simulink model "inverse_dynamic_control"  (R2017b)
settings: Solver=VariableStepAuto  StartTime=0.0  StopTime=3  RelTol=1e-3
InitFcn:
  | stop_time_as_str = get_param(gcs, 'StopTime');
  | stopTime = str2double(stop_time_as_str);
values from neighbouring files (symbols this model uses):
  KD = 50    [centralized_control_design.m]
  KP = 200    [centralized_control_design.m]
  max_torques = [56 97 52 10 10 10]    [centralized_control_design.m]
  min_torques = -[56 97 52 10 10 10]    [centralized_control_design.m]
libraries: roblocks x4
settings Model: Creator=jan  LastModifiedBy=jan.rosell

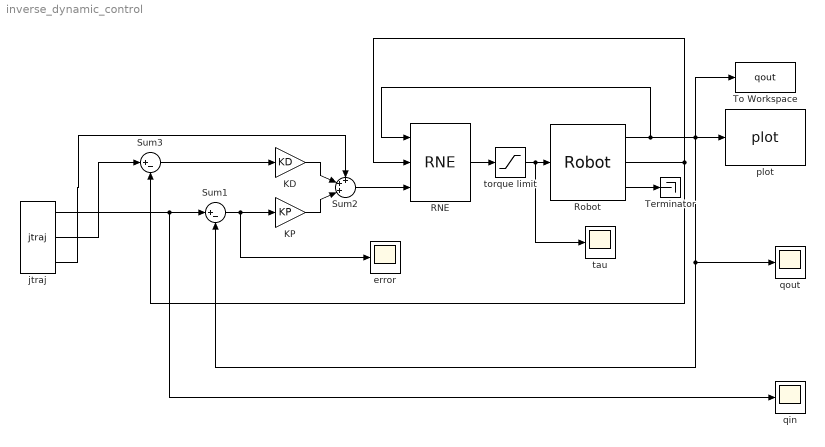
== system inverse_dynamic_control ==
  KD : Gain  Gain=KD
  KP : Gain  Gain=KP
  RNE : roblocks/Arm/RNE  robot=p560.nofriction  grav=[0 0 9.81]
  Robot : roblocks/Arm/Robot  robot=p560.nofriction  q0=[0 0 0 0 0 0]
  Sum1 : Sum  Inputs=|+-
  Sum2 : Sum  Inputs=+++|
  Sum3 : Sum  Inputs=|+-
  Terminator : Terminator
  To Workspace : ToWorkspace  VariableName=qout  SaveFormat=Timeseries  SampleTime=-1
  error : Scope
  jtraj : roblocks/Toolbox/jtraj  q0=[0 0 0 0 0 0]  qf=[pi/4 pi/2 -pi/2 0 0 0]  tmax=stopTime  ts=0.02
  plot : roblocks/Arm/plot  robot=p560  fps=10  holdplot=on
  qin : Scope
  qout : Scope
  tau : Scope
  torque limit : Saturate  UpperLimit=max_torques  LowerLimit=min_torques
  wires:
  Robot/3 -> Terminator/1
  Sum1/1 -> error/1, KP/1
  jtraj/1 -> qin/1, Sum1/1
  torque limit/1 -> tau/1, Robot/1
  RNE/1 -> torque limit/1
  Sum2/1 -> RNE/3
  Robot/1 -> RNE/1, To Workspace/1, plot/1, qout/1, Sum1/2
  Robot/2 -> Sum3/2, RNE/2
  KP/1 -> Sum2/3
  KD/1 -> Sum2/2
  jtraj/3 -> Sum2/1
  Sum3/1 -> KD/1
  jtraj/2 -> Sum3/1
